simulink model "LQR_simulink_Sily_test_fast"  (R2024b)
settings: Solver=ode4  StartTime=0.0  StopTime=5  FixedStep=0.005  RelTol=1e-3
values from neighbouring files (symbols this model uses):
  Ac = LinSystem.Ac    [LQR_client_Sily_test_fast.m]
  Bc = LinSystem.Bc    [LQR_client_Sily_test_fast.m]
  Cc = LinSystem.Cc    [LQR_client_Sily_test_fast.m]
  Dc = LinSystem.Dc    [LQR_client_Sily_test_fast.m]
  init_int_dref = -Ki_lqr\((Uinit-Us)+Kp_lqr*(Xinit_ss-Xs))    [LQR_client_Sily_test_fast.m]
  timestep = timeData.TimeStep    [LQR_client_Sily_test_fast.m]
undefined symbols (not defined in the file or in its folder): b_moment, Continuous, k_thrust, Ki_lqr, Kp_lqr, l, R_kalman, Time, Us, Xinit_ss, Xs
libraries: simulink_extras x6, ctrlSharedLib x1, simulink x1
settings Model: Creator=yaozhong.zhang  LastModifiedBy=Admin
settings DataIOCC: SaveOutput=off  SignalLogging=off  DSMLogging=off  SaveTime=off  ReturnWorkspaceOutputs=off
settings DebuggingCC: UnconnectedInputMsg=warning  UnconnectedOutputMsg=warning  UnconnectedLineMsg=warning
settings ModelReferenceCC: EnableRefExpFcnMdlSchedulingChecks=on
settings RTWCC: GPUComputeCapability=3.5

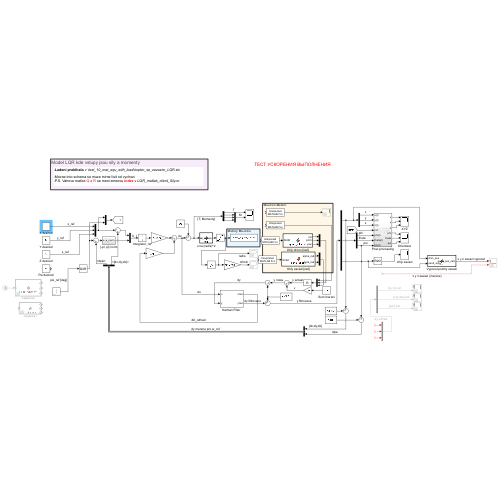
[thumbnail: Simulink's stored preview of the top-level diagram]
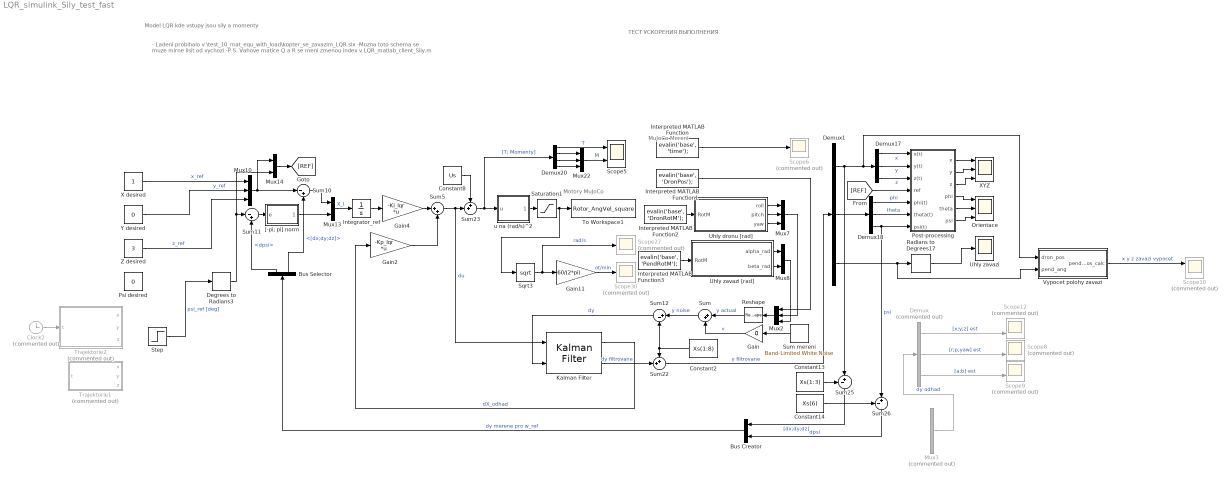
== system LQR_simulink_Sily_test_fast ==
  note: ТЕСТ УСКОРЕНИЯ ВЫПОЛНЕНИЯ
  note: Model LQR kde vstupy jsou sily a momenty
  note: MuJoCo Mereni
  note: - Ladeni probihalo v \test_10_mat_equ_with_load\kopter_se_zavazim_LQR.slx
      |
      | -Mozna toto schema se muze mirne lisit od vychozi
      | -P.S. Vahove matice Q a R se meni zmenou index v LQR_matlab_client_Sily.m
  note: Motory MuJoCo
  Bus Creator : BusCreator  Inputs=2
  Bus Selector : BusSelector  OutputSignals=dpsi,[dx;dy;dz]
  Clock2 : Clock  Commented=on
  Constant13 : Constant  Value=Xs(1:3)
  Constant14 : Constant  Value=Xs(6)
  Constant2 : Constant  Value=Xs(1:8)
  Constant8 : Constant  Value=Us
  Degrees to Radians3 : simulink_extras/Transformations/Degrees to Radians
  Demux : Demux  Commented=on  Outputs=3
  Demux1 : Demux  Outputs=3
  Demux17 : Demux  Outputs=3
  Demux18 : Demux  Outputs=3
  Demux20 : Demux
  Gain : Gain  Gain=0
  Gain11 : Gain  Gain=60/(2*pi)
  Gain2 : Gain  Gain=-Kp_lqr  Multiplication=Matrix(K*u)
  Gain4 : Gain  Gain=-Ki_lqr  Multiplication=Matrix(K*u)
  Integrator_ref : Integrator  InitialCondition=init_int_dref
  Interpreted MATLAB Function : MATLABFcn  MATLABFcn=evalin('base', 'time');
  Interpreted MATLAB Function1 : MATLABFcn  MATLABFcn=evalin('base', 'DronPos');  OutputDimensions=[3,1]  Output1D=off
  Interpreted MATLAB Function2 : MATLABFcn  MATLABFcn=evalin('base', 'DronRotM');  OutputDimensions=[3,3]  Output1D=off
  Interpreted MATLAB Function3 : MATLABFcn  MATLABFcn=evalin('base', 'PendRotM');  OutputDimensions=[3,3]  Output1D=off
  "Kalman Filter " : ctrlSharedLib/Kalman Filter  TimeDomain=Continuous-Time  UseCurrentEstimator=on  ModelSource=Individual A, B, C, D matrices  ModelSourceVariable=ss(0.95,1,1,0,1)  A=Ac  B=Bc  C=Cc  D=Dc  NumberOfStates=1  NumberOfInputs=1  NumberOfOutputs=1  InitialEstimateSource=Dialog  X0=Xinit_ss-Xs  P0=10  UseK=off  UseGH=off  NumberOfProcessNoiseInputs=1  G=1  TimeInvariantG=on  H=0  TimeInvariantH=on  Q=Q_kalman  TimeInvariantQ=on  R=R_kalman  TimeInvariantR=on  N=0  TimeInvariantN=on  AddInputPort=on  AddEnablePort=off  OutputEstimatedY=on  OutputP=off  Ts=-1
  Mux{2,7,10,22} (4 alike) : Mux  Inputs=3
  Mux13 : Mux  Inputs=2
  Mux14 : Mux  Inputs=2
  Mux3 : Mux  Commented=on  Inputs=3
  Mux8 : Mux  Inputs=2
  Orientace : Scope  NumInputPorts=3
  Post-processing : Subsystem
  Psi desired : Constant  Value=0
  Radians to Degrees17 : simulink_extras/Transformations/Radians to Degrees
  Reshape : Reshape  OutputDimensionality=Customize  OutputDimensions=[8,1]
  Saturation1 : Saturate  UpperLimit=1976^2  LowerLimit=0
  Scope{8..10,12} (4 alike) : Scope  Commented=on  NumInputPorts=2
  Scope27 : Scope  Commented=on
  Scope30 : Scope  Commented=on
  Scope5 : Scope  NumInputPorts=2
  Scope6 : Scope  Commented=on
  Sqrt3 : Sqrt
  Step : Step  Time=5  After=45  SampleTime=0
  Sum : Sum  Inputs=|++
  Sum mereni : simulink/Sources/Band-Limited White Noise  Cov=diag(R_kalman)*str2num(timestep)  Ts=str2num(timestep)  seed=[23341]
  Sum10 : Sum  Inputs=|-+
  Sum11 : Sum  Inputs=|-+
  Sum12 : Sum  Inputs=|+-
  Sum22 : Sum  Inputs=++|
  Sum23 : Sum  Inputs=++|
  Sum25 : Sum  Inputs=-+|
  Sum26 : Sum  Inputs=-+|
  Sum5 : Sum  Inputs=|++
  To Workspace1 : ToWorkspace  VariableName=Rotor_AngVel_square  SampleTime=-1
  Trajektorie1 : MATLAB Function  Commented=on  TreatAsAtomicUnit=on
  Trajektorie2 : MATLAB Function  Commented=on  TreatAsAtomicUnit=on
  Uhly dronu [rad] : MATLAB Function  TreatAsAtomicUnit=on
  Uhly zavazi : Scope
  Uhly zavazi [rad] : MATLAB Function  TreatAsAtomicUnit=on
  Vypocet polohy zavazi : MATLAB Function  TreatAsAtomicUnit=on
  X desired : Constant
  XYZ : Scope  NumInputPorts=3
  Y desired : Constant  Value=0
  Z desired : Constant  Value=3
  "[-pi; pi] norm" : Subsystem
  u na (rad/s)^2 : MATLAB Function  TreatAsAtomicUnit=on
  wires:
  Demux18/3 -> Post-processing/7(psi(t)), Sum26/2  "psi"
  u na (rad/s)^2/1(wi_square) -> Saturation1/1
  Demux/1 -> Scope12/2  "[x;y;z] est"
  Clock2/1 -> Trajektorie2/1(t)
  Sqrt3/1 -> Scope27/1, Gain11/1  "rad/s"
  ? -> Mux3/1
  Gain11/1 -> Scope30/1  "ot/min"
  Demux20/4 -> Mux22/3
  Sum5/1 -> "Kalman Filter "/1, Sum23/2  "du"
  Radians to Degrees17/1 -> Uhly zavazi/1
  Sum23/1 -> Demux20/1, u na (rad/s)^2/1(u)  "[T; Momenty]"
  Mux13/1 -> Integrator_ref/1  "X_I"
  Sum10/1 -> Mux13/1
  Sum26/1 -> Bus Creator/2  "dpsi"
  Uhly zavazi [rad]/2(beta_rad) -> Mux8/2
  Z desired/1 -> Mux10/3  "z_ref"
  ? -> Mux3/2
  Mux22/1 -> Scope5/2  "M"
  Bus Creator/1 -> Bus Selector/1  "dy merene pro w_ref"
  Step/1 -> Degrees to Radians3/1  "psi_ref [deg]"
  Interpreted MATLAB Function/1 -> Scope6/1
  Mux3/1 -> Demux/1  "dy odhad"
  Uhly zavazi [rad]/1(alpha_rad) -> Mux8/1
  X desired/1 -> Mux10/1  "x_ref"
  Uhly dronu [rad]/1(roll) -> Mux7/1
  Post-processing/6(psi) -> Orientace/3
  Post-processing/5(theta) -> Orientace/2
  Demux18/2 -> Post-processing/6(theta(t))  "theta"
  Sum11/1 -> "[-pi; pi] norm"/1(e)
  Y desired/1 -> Mux10/2  "y_ref"
  Demux18/1 -> Post-processing/5(phi(t))  "phi"
  Constant13/1 -> Sum25/1
  Constant14/1 -> Sum26/1
  Uhly dronu [rad]/2(pitch) -> Mux7/2
  Sum25/1 -> Bus Creator/1  "[dx;dy;dz]"
  Post-processing/4(phi) -> Orientace/1
  Bus Selector/1 -> Sum11/2  "<dpsi>"
  "[-pi; pi] norm"/1(e_norm) -> Mux13/2
  Integrator_ref/1 -> Gain4/1
  Bus Selector/2 -> Sum10/2  "<[dx;dy;dz]>"
  [REF] -> Post-processing/4(ref)
  Demux17/1 -> Post-processing/1(x(t))  "x"
  Mux14/1 -> [REF]
  Post-processing/2(y) -> XYZ/2
  Saturation1/1 -> Sqrt3/1, To Workspace1/1
  Demux17/2 -> Post-processing/2(y(t))  "y"
  Demux17/3 -> Post-processing/3(z(t))  "z"
  Demux20/1 -> Scope5/1  "T"
  "Kalman Filter "/1 -> Gain2/1  "dX_odhad"
  Degrees to Radians3/1 -> Mux14/2, Sum11/1
  Gain2/1 -> Sum5/2
  Demux20/2 -> Mux22/1
  Demux/2 -> Scope8/2  "[r;p;yaw] est"
  Post-processing/3(z) -> XYZ/3
  Constant8/1 -> Sum23/1
  Demux/3 -> Scope9/2  "[a;b] est"
  Mux10/1 -> Mux14/1, Sum10/1
  Gain4/1 -> Sum5/1
  Demux20/3 -> Mux22/2
  ? -> Mux3/3
  Post-processing/1(x) -> XYZ/1
  Uhly dronu [rad]/3(yaw) -> Mux7/3
  ? -> Scope10/2  "x y z zavazi (merene)"
  Interpreted MATLAB Function1/1 -> Mux2/1
  Mux7/1 -> Mux2/2
  Mux8/1 -> Mux2/3
  Mux2/1 -> Reshape/1
  Reshape/1 -> Sum/1  "y actual"
  Sum mereni/1 -> Gain/1
  Sum/1 -> Sum12/1  "y noise"
  Sum22/1 -> Demux1/1  "y filtrovane"
  "Kalman Filter "/2 -> Sum22/2  "dy filtrovane"
  Constant2/1 -> Sum22/1, Sum12/2
  Demux1/1 -> Vypocet polohy zavazi/1(dron_pos), Demux17/1, Sum25/2
  Demux1/2 -> Demux18/1
  Demux1/3 -> Vypocet polohy zavazi/2(pend_ang), Radians to Degrees17/1
  Sum12/1 -> "Kalman Filter "/2  "dy"
  Gain/1 -> Sum/2  "v"
  Vypocet polohy zavazi/1(pend_pos_calc) -> Scope10/1  "x y z zavazi vypocet"
  Interpreted MATLAB Function2/1 -> Uhly dronu [rad]/1(RotM)
  Interpreted MATLAB Function3/1 -> Uhly zavazi [rad]/1(RotM)

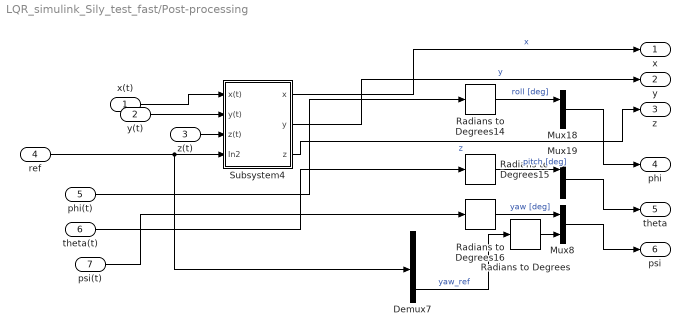
== system LQR_simulink_Sily_test_fast/Post-processing ==
  x(t) : Inport
  y(t) : Inport  Port=2
  z(t) : Inport  Port=3
  ref : Inport  Port=4
  phi(t) : Inport  Port=5
  theta(t) : Inport  Port=6
  psi(t) : Inport  Port=7
  Demux7 : Demux
  Mux18 : Mux  Inputs=2
  Mux19 : Mux  Inputs=2
  Mux8 : Mux  Inputs=2
  Radians to Degrees{,14..16} (4 alike) : simulink_extras/Transformations/Radians to Degrees
  Subsystem4 : Subsystem
  x : Outport
  y : Outport  Port=2
  z : Outport  Port=3
  phi : Outport  Port=4
  theta : Outport  Port=5
  psi : Outport  Port=6
  wires:
  Radians to Degrees16/1 -> Mux8/1  "yaw [deg]"
  ref/1 -> Subsystem4/4(In2), Demux7/1
  Demux7/4 -> Radians to Degrees/1  "yaw_ref"
  theta(t)/1 -> Radians to Degrees15/1
  Mux18/1 -> phi/1
  Subsystem4/3(z) -> z/1  "z"
  Radians to Degrees14/1 -> Mux18/1  "roll [deg]"
  Radians to Degrees15/1 -> Mux19/1  "pitch [deg]"
  Subsystem4/2(y) -> y/1  "y"
  x(t)/1 -> Subsystem4/1(x(t))
  y(t)/1 -> Subsystem4/2(y(t))
  psi(t)/1 -> Radians to Degrees16/1
  phi(t)/1 -> Radians to Degrees14/1
  Subsystem4/1(x) -> x/1  "x"
  Mux8/1 -> psi/1
  z(t)/1 -> Subsystem4/3(z(t))
  Mux19/1 -> theta/1
  Radians to Degrees/1 -> Mux8/2

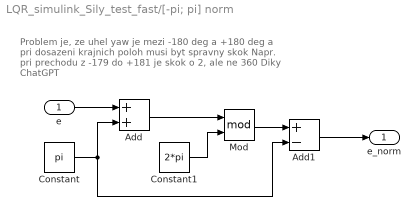
== system LQR_simulink_Sily_test_fast/[-pi; pi] norm ==
  note: Problem je, ze uhel yaw je mezi -180 deg a +180 deg
      | a pri dosazeni krajnich poloh musi byt spravny skok
      | Napr. pri prechodu z -179 do +181 je skok o 2, ale ne 360
      | Diky ChatGPT
  e : Inport
  Add : Sum
  Add1 : Sum  Inputs=+-
  Constant : Constant  Value=pi
  Constant1 : Constant  Value=2*pi
  Mod : Math  Operator=mod
  e_norm : Outport
  wires:
  e/1 -> Add/1
  Add/1 -> Mod/1
  Constant/1 -> Add1/2, Add/2
  Constant1/1 -> Mod/2
  Mod/1 -> Add1/1
  Add1/1 -> e_norm/1

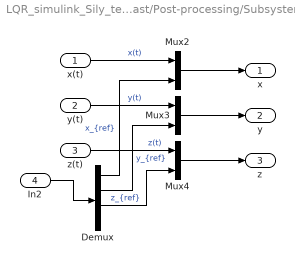
== system LQR_simulink_Sily_test_fast/Post-processing/Subsystem4 ==
  x(t) : Inport
  y(t) : Inport  Port=2
  z(t) : Inport  Port=3
  In2 : Inport  Port=4
  Demux : Demux
  Mux2 : Mux  Inputs=2
  Mux3 : Mux  Inputs=2
  Mux4 : Mux  Inputs=2
  x : Outport
  y : Outport  Port=2
  z : Outport  Port=3
  wires:
  Demux/2 -> Mux3/2  "y_{ref}"
  Mux4/1 -> z/1
  y(t)/1 -> Mux3/1  "y(t)"
  Mux3/1 -> y/1
  Demux/1 -> Mux2/2  "x_{ref}"
  Demux/3 -> Mux4/2  "z_{ref}"
  Mux2/1 -> x/1
  In2/1 -> Demux/1
  x(t)/1 -> Mux2/1  "x(t)"
  z(t)/1 -> Mux4/1  "z(t)"

== matlab function LQR_simulink_Sily_test_fast/Trajektorie1 ==
  data: x output; t input; y output; z output
function [x, y, z] = Trajectory(t)
% t — текущее время симуляции (0–60 секунд)
% x, y, z — координаты объекта

% Параметры
t_total = 60;              % общее время
t_phase1 = 7;              % время фазы 1 (разгон по X)
spiral_radius = 4;         % радиус спирали
z_start = 2;
z_end = 10;
z_per_turn = 2;
n_turns = (z_end - z_start) / z_per_turn;
t_spiral = t_total - t_phase1;   % длительность спирали
omega = 2*pi*n_turns / t_spiral; % угловая скорость

if t <= t_phase1
    % Фаза 1: прямое движение по X от 0 до 2
    x = 2 * (t / t_phase1);
    y = 0;
    z = z_start;
else
    % Фаза 2: движение по спирали
    t2 = t - t_phase1;
    theta = omega * t2;

    x = spiral_radius * cos(theta);
    y = spiral_radius * sin(theta);
    z = z_start + (z_end - z_start) * (t2 / t_spiral);
end
end

== matlab function LQR_simulink_Sily_test_fast/Vypocet polohy zavazi ==
  data: pend_pos_calc output; dron_pos input; pend_ang input; d parameter
function pend_pos_calc = fcn(dron_pos, pend_ang, d)
% pro kontrolu vypocetu polohu zavazi z uhlu a polohy dronu

x = dron_pos(1);
y = dron_pos(2);
z = dron_pos(3);

alpha = pend_ang(1);
beta = pend_ang(2);

x_d = x + d*cos(beta)*sin(alpha);
y_d = y + d*sin(beta);
z_d = z - d*cos(beta)*cos(alpha);

pend_pos_calc = [x_d; y_d; z_d];

== matlab function LQR_simulink_Sily_test_fast/Trajektorie2 ==
  data: x output; t input; y output; z output
function [x, y, z] = spiralTrajectory(t)
% t — текущее время симуляции (0–60 секунд)
% x, y, z — координаты объекта

% Параметры
t_total = 60;              % общее время
t_phase1 = 7;              % время фазы 1 (разгон по X)
spiral_radius = 4;         % радиус спирали
z_start = 2;
z_end = 10;
z_per_turn = 2;
n_turns = (z_end - z_start) / z_per_turn;
t_spiral = t_total - t_phase1;   % длительность спирали
omega = 2*pi*n_turns / t_spiral; % угловая скорость

if t <= t_phase1
    % Фаза 1: прямое движение по X от 0 до 2
    x = 2 * (t / t_phase1);
    y = 0;
    z = z_start;
else
    % Фаза 2: движение по спирали
    t2 = t - t_phase1;
    theta = omega * t2;

    x = spiral_radius * cos(theta);
    y = spiral_radius * sin(theta);
    z = z_start + (z_end - z_start) * (t2 / t_spiral);
end
end

== matlab function LQR_simulink_Sily_test_fast/Uhly dronu [rad] ==
  data: RotM input; roll output; pitch output; yaw output
function [roll, pitch, yaw] = quad_attitude(RotM)
% matice rotace koptery z Python, vuci svetu!!!
% rotm2eul prevadi na Eulerove uhly
radians = rotm2eul(RotM, 'ZYX'); % pouzivam poradi ZYX

% roll = kolem x, pitch = kolem y, yaw = kolem z
yaw = radians(1);
pitch = radians(2);
roll = radians(3);
end

== matlab function LQR_simulink_Sily_test_fast/Uhly zavazi [rad] ==
  data: RotM input; alpha_rad output; beta_rad output
function [alpha_rad, beta_rad] = pend_orient(RotM)
% Расчет углов альфа и бета маятника

% Вектор маятника
rope_vector = RotM * [0; 0; -1];

% Расчет угла альфа
rope_vector_xz = rope_vector([1, 3]); % Компоненты x и z
z_axis = [0; -1];
cos_alpha = dot(rope_vector_xz, z_axis) / (norm(rope_vector_xz) * norm(z_axis));
cos_alpha = max(-1, min(1, cos_alpha)); % Ограничиваем в диапазоне [-1, 1]
alpha = acos(cos_alpha);
if rope_vector(1) < 0
    alpha = -alpha;
end

% Расчет угла бета
rope_vector_xz_3 = [rope_vector(1); 0; rope_vector(3)];
cos_beta = dot(rope_vector, rope_vector_xz_3) / (norm(rope_vector) * norm(rope_vector_xz_3));
cos_beta = max(-1, min(1, cos_beta)); % Ограничиваем в диапазоне [-1, 1]
beta = acos(cos_beta);
if rope_vector(2) < 0
    beta = -beta;
end

% Округляем до 5 знаков после запятой
% alpha_rad = round(alpha, 5); %[rad]
% beta_rad = round(beta, 5); %[rad]
alpha_rad = alpha;
beta_rad = beta;

== matlab function LQR_simulink_Sily_test_fast/u na (rad//s)^2 ==
  data: u input; wi_square output; b_moment parameter; k_thrust parameter; l parameter
function wi_square = fcn(u, b_moment, k_thrust, l)

T = u(1);
Tau_phi = u(2);
Tau_theta = u(3);
Tau_psi = u(4);

w1 = ( (Tau_phi*b_moment - Tau_theta*b_moment + l*T*b_moment + l*Tau_psi*k_thrust)/(4*l*b_moment*k_thrust));
w2 = ( (-Tau_theta*b_moment - Tau_phi*b_moment + l*T*b_moment - l*Tau_psi*k_thrust)/(4*l*b_moment*k_thrust));
w3 = ( (Tau_theta*b_moment - Tau_phi*b_moment + l*T*b_moment + l*Tau_psi*k_thrust)/(4*l*b_moment*k_thrust));
w4 = ( (Tau_phi*b_moment + Tau_theta*b_moment + l*T*b_moment - l*Tau_psi*k_thrust)/(4*l*b_moment*k_thrust));

wi_square = [w1;w2;w3;w4];
